simulink model "validation_network_armax_y1y2y3"  (R2024a)
settings: Solver=FixedStepDiscrete  StartTime=0.0  StopTime=499  FixedStep=1  RelTol=1e-3
values from neighbouring files (symbols this model uses):
  theta = [1 0.25 0.3 0.15 0.3 -0.01 -0.8 0.15 0.8 -0.3 -0.8 0.2 ... (42 elements, 1x42)]    [Copy_of_true_system.mat]    (also in a_generate_stable_system.m = [A1(2:3)' B1' C1(2:3)' A2(2:3)' B2' C2(2:3)' A3(2:3)' B3' C3)
settings Model: Creator=jogal  LastModifiedBy=jogal
settings OptimizationCC: ReuseModelBlockBuffer=off
settings RTWCC: GPUComputeCapability=3.5

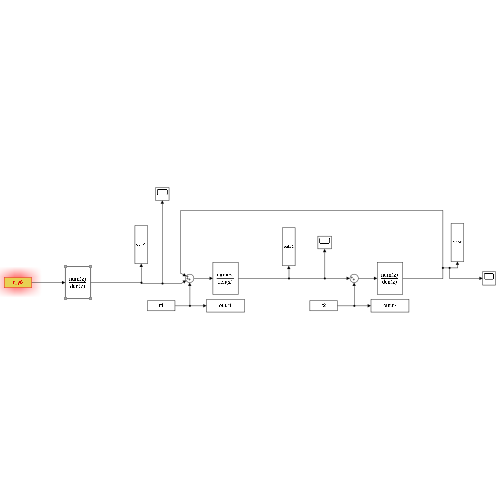
[thumbnail: Simulink's stored preview of the top-level diagram]
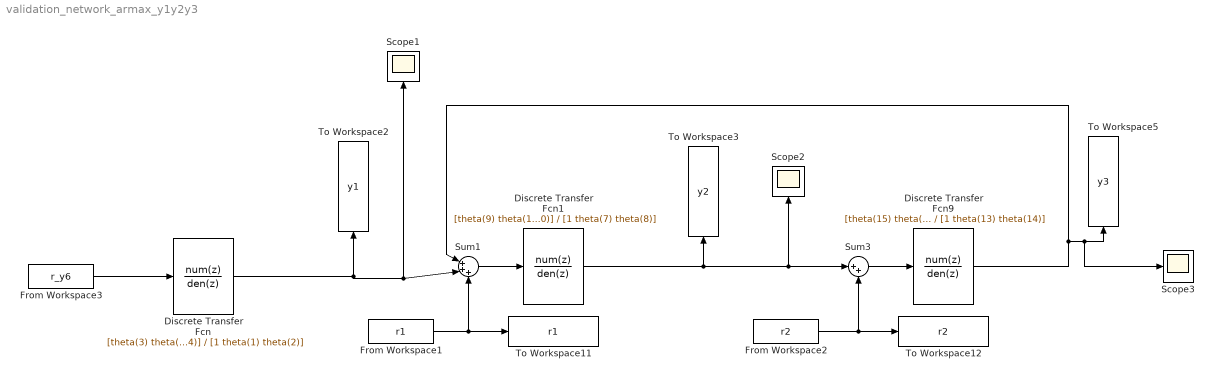
== system validation_network_armax_y1y2y3 ==
  Discrete Transfer Fcn : DiscreteTransferFcn  Numerator=[theta(3) theta(4)]  Denominator=[1 theta(1) theta(2)]
  Discrete Transfer Fcn1 : DiscreteTransferFcn  Numerator=[theta(9) theta(10)]  Denominator=[1 theta(7) theta(8)]
  Discrete Transfer Fcn9 : DiscreteTransferFcn  Numerator=[theta(15) theta(16)]  Denominator=[1 theta(13) theta(14)]
  From Workspace1 : FromWorkspace  VariableName=r1  SampleTime=1  Interpolate=off  OutputAfterFinalValue=Holding final value
  From Workspace2 : FromWorkspace  VariableName=r2  SampleTime=1  Interpolate=off  OutputAfterFinalValue=Holding final value
  From Workspace3 : FromWorkspace  VariableName=r_y6  SampleTime=1  Interpolate=off  OutputAfterFinalValue=Holding final value
  Scope1 : Scope
  Scope2 : Scope
  Scope3 : Scope
  Sum1 : Sum  Inputs=|+++
  Sum3 : Sum  Inputs=|++
  To Workspace11 : ToWorkspace  VariableName=r1  SampleTime=-1
  To Workspace12 : ToWorkspace  VariableName=r2  SampleTime=-1
  To Workspace2 : ToWorkspace  VariableName=y1  SampleTime=-1
  To Workspace3 : ToWorkspace  VariableName=y2  SampleTime=-1
  To Workspace5 : ToWorkspace  VariableName=y3  SampleTime=-1
  wires:
  From Workspace1/1 -> Sum1/3, To Workspace11/1
  Sum1/1 -> Discrete Transfer Fcn1/1
  From Workspace2/1 -> To Workspace12/1, Sum3/2
  Sum3/1 -> Discrete Transfer Fcn9/1
  Discrete Transfer Fcn9/1 -> Sum1/1, Scope3/1, To Workspace5/1
  Discrete Transfer Fcn/1 -> To Workspace2/1, Scope1/1, Sum1/2
  Discrete Transfer Fcn1/1 -> Sum3/1, Scope2/1, To Workspace3/1
  From Workspace3/1 -> Discrete Transfer Fcn/1
